simulink model "conversionYUV"  (R2018b)
settings: Solver=ode3  StartTime=0  StopTime=TFinal  FixedStep=0.2  RelTol=1e-3  EnableMultiTasking=on
settings Model: ExtModeTrigDuration=80  Creator=The MathWorks, Inc.  LastModifiedBy=taodu
settings DataIOCC: LimitDataPoints=on  SaveFormat=StructureWithTime  SaveOutput=off  SaveTime=off
settings OptimizationCC: BlockReduction=off  EnhancedBackFolding=on  PassReuseOutputArgsAs=Individual arguments  MaxStackSize=64  OptimizeBlockOrder=speed  DifferentSizesBufferReuse=on  OptimizationCustomize=off
settings DebuggingCC: AlgebraicLoopMsg=none  ParameterPrecisionLossMsg=none  ParameterTunabilityLossMsg=error  UnconnectedInputMsg=none  UnconnectedOutputMsg=none  UnconnectedLineMsg=none  BusObjectLabelMismatch=error  LibraryContextMissingDiagnostic=none  SFUnexpectedBacktrackingDiag=warning  SFNoUnconditionalDefaultTransitionDiag=warning  SFExecutionAtInitializationDiag=none
settings HardwareCC: ProdBitPerPointer=32  ProdBitPerSizeT=32  ProdBitPerPtrDiffT=32  ProdLargestAtomicInteger=Long  ProdWordSize=32  ProdHWDeviceType=ARM Compatible->ARM 9  UseEmbeddedCoderFeatures=off
settings ModelReferenceCC: PropagateSignalLabelsOutOfModel=off
settings SFSimCC: SimUseLocalCustomCode=off  MATLABDynamicMemAlloc=off
settings RTWCC: SystemTargetFile=ert.tlc  HardwareBoard=PARROT Rolling Spider  TemplateMakefile=ert_default_tmf  GenerateReport=on  RTWUseLocalCustomCode=off  Toolchain=Sourcery G++ Lite GNU Toolchain for Drones  IncludeHyperlinkInReport=on  LaunchReport=on  GenerateTraceInfo=on  GenerateTraceReport=on  GenerateTraceReportSl=on  GenerateTraceReportSf=on  GenerateTraceReportEml=on
settings CodeAppCC: ForceParamTrailComments=on  IgnoreCustomStorageClasses=off  MaxIdLength=63  OperatorAnnotations=on  SimulinkDataObjDesc=on  SFDataObjDesc=on  InsertBlockDesc=on
settings ERTTargetCC: MatFileLogging=on  SupportNonInlinedSFcns=on
settings ConfigComp: CovMetricSettings=dw  CovHtmlReporting=on  CovSaveCumulativeToWorkspaceVar=on  CovSaveSingleToWorkspaceVar=on  CovExternalEMLEnable=off  CovSFcnEnable=off

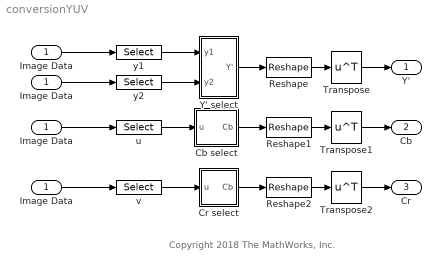
== system conversionYUV ==
  note: Copyright 2018 The MathWorks, Inc.
  Image Data : Inport  OutDataTypeStr=uint8  PortDimensions=[4 9600]  SampleTime=[0.20000000000000001,0]
  " Image Data " : InportShadow  OutDataTypeStr=uint8  PortDimensions=[4 9600]  SampleTime=[0.20000000000000001,0]
  Cb select : Subsystem
  Cr select : Subsystem
  "Image Data " : InportShadow  OutDataTypeStr=uint8  PortDimensions=[4 9600]  SampleTime=[0.20000000000000001,0]
  "Image Data  " : InportShadow  OutDataTypeStr=uint8  PortDimensions=[4 9600]  SampleTime=[0.20000000000000001,0]
  Reshape : Reshape  OutputDimensionality=Customize  OutputDimensions=[160 120]
  Reshape1 : Reshape  OutputDimensionality=Customize  OutputDimensions=[160 120]
  Reshape2 : Reshape  OutputDimensionality=Customize  OutputDimensions=[160 120]
  Transpose : Math  Operator=transpose  SaturateOnIntegerOverflow=on
  Transpose1 : Math  Operator=transpose  SaturateOnIntegerOverflow=on
  Transpose2 : Math  Operator=transpose  SaturateOnIntegerOverflow=on
  Y' select : Subsystem
  u : Selector  NumberOfDimensions=2  InputPortWidth=3  IndexOptions=Index vector (dialog),Select all  Indices=2,1  OutputSizes=1,1
  v : Selector  NumberOfDimensions=2  InputPortWidth=3  IndexOptions=Index vector (dialog),Select all  Indices=4,1  OutputSizes=1,1
  y1 : Selector  NumberOfDimensions=2  InputPortWidth=3  IndexOptions=Index vector (dialog),Select all  Indices=1,1  OutputSizes=1,1
  y2 : Selector  NumberOfDimensions=2  InputPortWidth=3  IndexOptions=Index vector (dialog),Select all  Indices=3,1  OutputSizes=1,1
  Y' : Outport  OutDataTypeStr=uint8  PortDimensions=[120 160]
  Cb : Outport  Port=2  OutDataTypeStr=uint8  PortDimensions=[120 160]
  Cr : Outport  Port=3  OutDataTypeStr=uint8  PortDimensions=[120 160]
  wires:
  Transpose2/1 -> Cr/1
  y1/1 -> Y' select/1(y1)
  Reshape2/1 -> Transpose2/1
  Y' select/1(Y') -> Reshape/1
  Cr select/1(Cb) -> Reshape2/1
  y2/1 -> Y' select/2(y2)
  Reshape1/1 -> Transpose1/1
  u/1 -> Cb select/1(u)
  v/1 -> Cr select/1(u)
  Transpose1/1 -> Cb/1
  Cb select/1(Cb) -> Reshape1/1
  Reshape/1 -> Transpose/1
  Transpose/1 -> Y'/1
  "Image Data "/1 -> u/1
  " Image Data "/1 -> v/1
  Image Data/1 -> y2/1
  "Image Data  "/1 -> y1/1

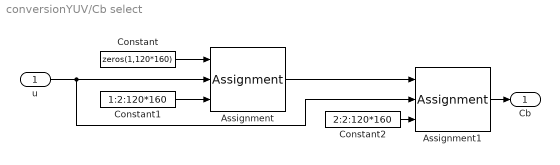
== system conversionYUV/Cb select ==
  u : Inport
  Assignment : Assignment  DiagnosticForDimensions=Warning  IndexOptions=Index vector (port)  Indices=1  OutputSizes=1
  Assignment1 : Assignment  DiagnosticForDimensions=Warning  IndexOptions=Index vector (port)  Indices=1  OutputSizes=1
  Constant : Constant  Value=zeros(1,120*160)  OutDataTypeStr=uint8
  Constant1 : Constant  Value=1:2:120*160
  Constant2 : Constant  Value=2:2:120*160
  Cb : Outport
  wires:
  Constant2/1 -> Assignment1/3
  Constant1/1 -> Assignment/3
  Constant/1 -> Assignment/1
  Assignment1/1 -> Cb/1
  u/1 -> Assignment/2, Assignment1/2
  Assignment/1 -> Assignment1/1

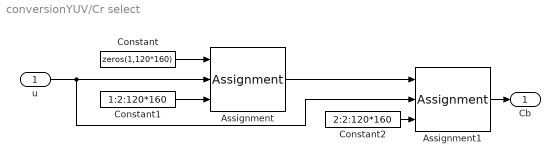
== system conversionYUV/Cr select ==
  u : Inport
  Assignment : Assignment  DiagnosticForDimensions=Warning  IndexOptions=Index vector (port)  Indices=1  OutputSizes=1
  Assignment1 : Assignment  DiagnosticForDimensions=Warning  IndexOptions=Index vector (port)  Indices=1  OutputSizes=1
  Constant : Constant  Value=zeros(1,120*160)  OutDataTypeStr=uint8
  Constant1 : Constant  Value=1:2:120*160
  Constant2 : Constant  Value=2:2:120*160
  Cb : Outport
  wires:
  Assignment/1 -> Assignment1/1
  u/1 -> Assignment1/2, Assignment/2
  Assignment1/1 -> Cb/1
  Constant/1 -> Assignment/1
  Constant1/1 -> Assignment/3
  Constant2/1 -> Assignment1/3

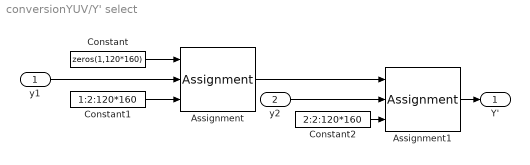
== system conversionYUV/Y' select ==
  y1 : Inport
  y2 : Inport  Port=2
  Assignment : Assignment  DiagnosticForDimensions=Warning  IndexOptions=Index vector (port)  Indices=1  OutputSizes=1
  Assignment1 : Assignment  DiagnosticForDimensions=Warning  IndexOptions=Index vector (port)  Indices=1  OutputSizes=1
  Constant : Constant  Value=zeros(1,120*160)  OutDataTypeStr=uint8
  Constant1 : Constant  Value=1:2:120*160
  Constant2 : Constant  Value=2:2:120*160
  Y' : Outport
  wires:
  y1/1 -> Assignment/2
  Assignment/1 -> Assignment1/1
  y2/1 -> Assignment1/2
  Assignment1/1 -> Y'/1
  Constant/1 -> Assignment/1
  Constant1/1 -> Assignment/3
  Constant2/1 -> Assignment1/3
